simulink model "FirstOrderSystem_wDelay_KF"  (R2020b)
settings: Solver=ode4  StartTime=0.0  StopTime=SIM_TIME  FixedStep=STEP_SIZE  RelTol=1e-3
values from neighbouring files (symbols this model uses):
  A = alpha    (= -1)    [FirstOrderSystem_wDelay_KF_init.m]
  A_kf = [A B*Ctau;zeros(2,1) Atau]    [FirstOrderSystem_wDelay_KF_init.m]
  B = 1    [FirstOrderSystem_wDelay_KF_init.m]
  B_kf = [B*Dtau; Btau]    [FirstOrderSystem_wDelay_KF_init.m]
  C = 1    [FirstOrderSystem_wDelay_KF_init.m]
  C_kf = [C zeros(1,2)]    [FirstOrderSystem_wDelay_KF_init.m]
  D = 0    [FirstOrderSystem_wDelay_KF_init.m]
  STEP_SIZE = 0.01    [FirstOrderSystem_wDelay_KF_init.m]
  T = tau(4)    [FirstOrderSystem_wDelay_KF_init.m]
  Tc = 0.01    [FirstOrderSystem_wDelay_KF_init.m]
  x0 = 20    [FirstOrderSystem_wDelay_KF_init.m]
  xhat0 = zeros(3,1)    [FirstOrderSystem_wDelay_KF_init.m]
undefined symbols (not defined in the file or in its folder): L, square
libraries: simulink x2
settings Model: Creator=Roberto  LastModifiedBy=roga
settings DataIOCC: ReturnWorkspaceOutputs=off
settings DebuggingCC: ArithmeticOperatorsInVariantConditions=warning
settings SFSimCC: SimUseLocalCustomCode=off  CustomCodeUndefinedFunction=UseInterfaceOnly
settings RTWCC: RTWUseLocalCustomCode=off

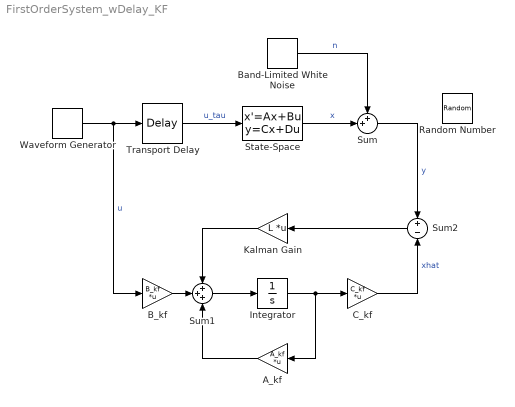
== system FirstOrderSystem_wDelay_KF ==
  A_kf : Gain  Gain=A_kf  Multiplication=Matrix(K*u) (u vector)
  B_kf : Gain  Gain=B_kf  Multiplication=Matrix(K*u) (u vector)
  Band-Limited White Noise : simulink/Sources/Band-Limited White Noise  Cov=Vn  Ts=Tc  seed=[23341]
  C_kf : Gain  Gain=C_kf  Multiplication=Matrix(K*u) (u vector)
  Integrator : Integrator  InitialCondition=xhat0
  Kalman Gain : Gain  Gain=L  Multiplication=Matrix(K*u) (u vector)
  Random Number : RandomNumber  SampleTime=0.1
  State-Space : StateSpace  A=A  B=B  C=C  D=D  InitialCondition=x0
  Sum : Sum  Inputs=++|
  Sum1 : Sum  Inputs=+++
  Sum2 : Sum  Inputs=+-
  Transport Delay : TransportDelay  DelayTime=T
  Waveform Generator : simulink/Sources/Waveform Generator  OutMin=[]  OutMax=[]  OutDataTypeStr=double  SelectedSignal=1  Signals=square(10,2*pi/5,0,50)  BlockNames=MultiportSwitch_6ce1bd8383e244b  SampleTime=STEP_SIZE
  wires:
  Transport Delay/1 -> State-Space/1  "u_tau"
  State-Space/1 -> Sum/2  "x"
  Band-Limited White Noise/1 -> Sum/1  "n"
  Waveform Generator/1 -> B_kf/1, Transport Delay/1  "u"
  Sum/1 -> Sum2/1  "y"
  Sum1/1 -> Integrator/1
  Kalman Gain/1 -> Sum1/1
  Sum2/1 -> Kalman Gain/1
  C_kf/1 -> Sum2/2  "xhat"
  B_kf/1 -> Sum1/2
  Integrator/1 -> C_kf/1, A_kf/1
  A_kf/1 -> Sum1/3
